simulink model "WhirlyBird_PD"  (R2016b)
settings: Solver=ode45  StartTime=0.0  StopTime=10000  RelTol=1e-3  EnableMultiTasking=on
InitFcn:
  | param
undefined symbols (not defined in the file or in its folder): drawWhirly, P, whirly_ctrl
settings Model: Creator=beard  LastModifiedBy=Jacob
settings DataIOCC: LimitDataPoints=on  SaveFormat=Array  SignalLoggingSaveFormat=ModelDataLogs
settings OptimizationCC: ExpressionDepthLimit=2147483647  InitFltsAndDblsToZero=on  LifeSpan=inf
settings DebuggingCC: UnderspecifiedInitializationDetection=Classic  MergeDetectMultiDrivingBlocksExec=none  SolverPrmCheckMsg=warning  FcnCallInpInsideContextMsg=warning  StateNameClashWarn=warning  SFUnexpectedBacktrackingDiag=warning  SFNoUnconditionalDefaultTransitionDiag=warning  SFExecutionAtInitializationDiag=none
settings HardwareCC: ProdBitPerPointer=32  ProdBitPerSizeT=32  ProdBitPerPtrDiffT=32  ProdLargestAtomicFloat=None  ProdIntDivRoundTo=Undefined  ProdEndianess=Unspecified  ProdWordSize=32  ProdHWDeviceType=32-bit Generic
settings ModelReferenceCC: PropagateSignalLabelsOutOfModel=off
settings GRTTargetCC: TargetLangStandard=C89/C90 (ANSI)  GeneratePreprocessorConditionals=Disable all  CombineOutputUpdateFcns=off  GRTInterface=on
settings ConfigComp: CovMetricSettings=dw  CovHtmlReporting=on  CovSaveCumulativeToWorkspaceVar=on  CovSaveSingleToWorkspaceVar=on  CovExternalEMLEnable=off

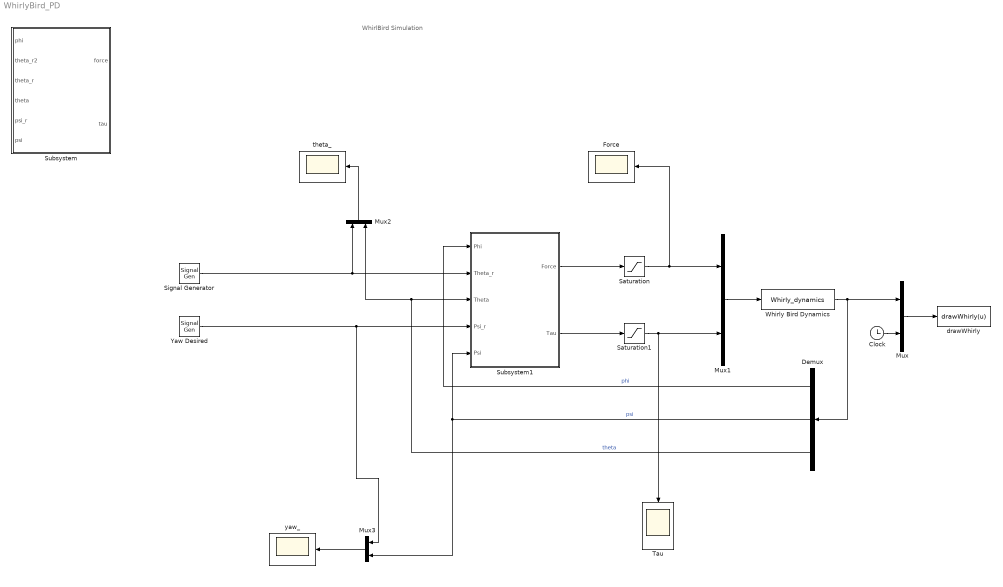
== system WhirlyBird_PD ==
  note: WhirlBird Simulation
  Clock : Clock
  Demux : Demux  Outputs=3
  Force : Scope
  Mux{,1..3} (4 alike) : Mux  Inputs=2
  Saturation : Saturate  UpperLimit=P.Fmax  LowerLimit=0
  Saturation1 : Saturate  UpperLimit=P.Taumax  LowerLimit=-P.Taumax
  Signal Generator : SignalGenerator  WaveForm=square  Amplitude=.2618*2  Frequency=.02
  Subsystem : Subsystem
  Subsystem1 : Subsystem
  Tau : Scope
  Whirly Bird Dynamics : S-Function  FunctionName=Whirly_dynamics  Parameters=P  SFunctionDeploymentMode=off  EnableBusSupport=off
  Yaw Desired : SignalGenerator  WaveForm=square  Amplitude=.2618*2  Frequency=.02
  drawWhirly : MATLABFcn  MATLABFcn=drawWhirly(u)  OutputDimensions=0  SampleTime=0.1
  theta_ : Scope
  yaw_ : Scope
  wires:
  Whirly Bird Dynamics/1 -> Mux/1, Demux/1
  Clock/1 -> Mux/2
  Mux/1 -> drawWhirly/1
  Signal Generator/1 -> Subsystem1/2(Theta_r), Mux2/1
  Mux2/1 -> theta_/1
  Mux1/1 -> Whirly Bird Dynamics/1
  Demux/3 -> Mux2/2, Subsystem1/3(Theta)  "theta"
  Saturation/1 -> Force/1, Mux1/1
  Demux/2 -> Subsystem1/5(Psi), Mux3/2  "psi"
  Yaw Desired/1 -> Mux3/1, Subsystem1/4(Psi_r)
  Mux3/1 -> yaw_/1
  Saturation1/1 -> Mux1/2, Tau/1
  Demux/1 -> Subsystem1/1(Phi)  "phi"
  Subsystem1/1(Force) -> Saturation/1
  Subsystem1/2(Tau) -> Saturation1/1

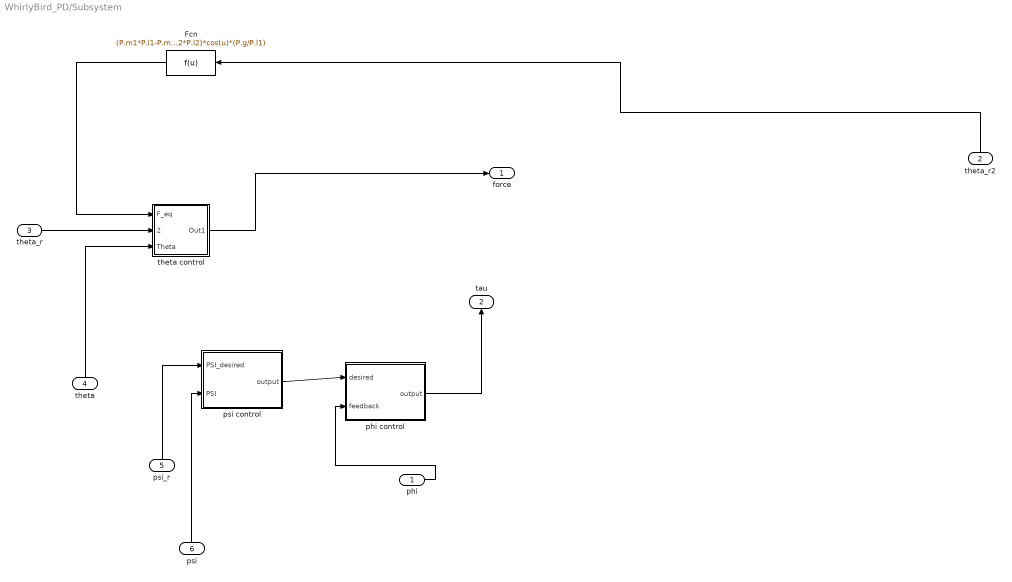
== system WhirlyBird_PD/Subsystem ==
  phi : Inport
  theta_r2 : Inport  Port=2
  theta_r : Inport  Port=3
  theta : Inport  Port=4
  psi_r : Inport  Port=5
  psi : Inport  Port=6
  Fcn : Fcn  Expr=(P.m1*P.l1-P.m2*P.l2)*cos(u)*(P.g/P.l1)
  phi control : Subsystem
  psi control : Subsystem
  theta control : Subsystem
  force : Outport
  tau : Outport  Port=2
  wires:
  theta/1 -> theta control/3(Theta)
  theta_r/1 -> theta control/2(Theta_d)
  theta_r2/1 -> Fcn/1
  psi/1 -> psi control/2(PSI)
  psi_r/1 -> psi control/1(PSI_desired)
  phi/1 -> phi control/2(feedback)
  phi control/1(output) -> tau/1
  theta control/1(Out1) -> force/1
  Fcn/1 -> theta control/1(F_eq)
  psi control/1(output) -> phi control/1(desired)

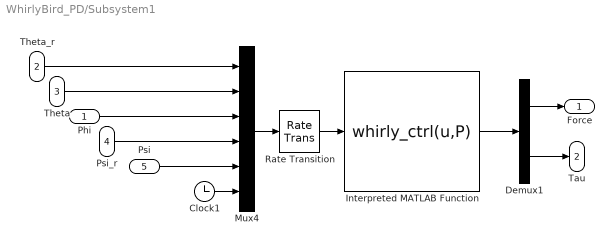
== system WhirlyBird_PD/Subsystem1 ==
  Phi : Inport
  Theta_r : Inport  Port=2
  Theta : Inport  Port=3
  Psi_r : Inport  Port=4
  Psi : Inport  Port=5
  Clock1 : Clock
  Demux1 : Demux  Outputs=2
  Interpreted MATLAB Function : MATLABFcn  MATLABFcn=whirly_ctrl(u,P)  OutputDimensions=2
  Mux4 : Mux  Inputs=6
  Rate Transition : RateTransition  OutPortSampleTime=P.Ts
  Force : Outport
  Tau : Outport  Port=2
  wires:
  Theta_r/1 -> Mux4/1
  Psi/1 -> Mux4/5
  Psi_r/1 -> Mux4/4
  Theta/1 -> Mux4/2
  Clock1/1 -> Mux4/6
  Phi/1 -> Mux4/3
  Rate Transition/1 -> Interpreted MATLAB Function/1
  Mux4/1 -> Rate Transition/1
  Interpreted MATLAB Function/1 -> Demux1/1
  Demux1/1 -> Force/1
  Demux1/2 -> Tau/1

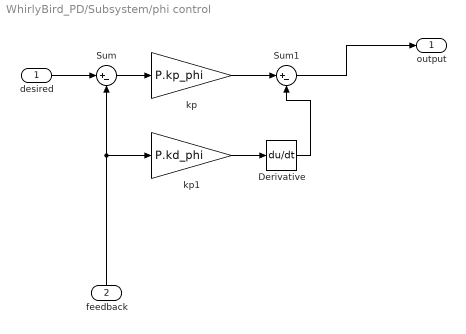
== system WhirlyBird_PD/Subsystem/phi control ==
  desired : Inport
  feedback : Inport  Port=2
  Derivative : Derivative
  Sum : Sum  Inputs=|+-
  Sum1 : Sum  Inputs=|+-
  kp : Gain  Gain=P.kp_phi
  kp1 : Gain  Gain=P.kd_phi
  output : Outport
  wires:
  desired/1 -> Sum/1
  feedback/1 -> kp1/1, Sum/2
  Sum1/1 -> output/1
  kp1/1 -> Derivative/1
  Sum/1 -> kp/1
  kp/1 -> Sum1/1
  Derivative/1 -> Sum1/2

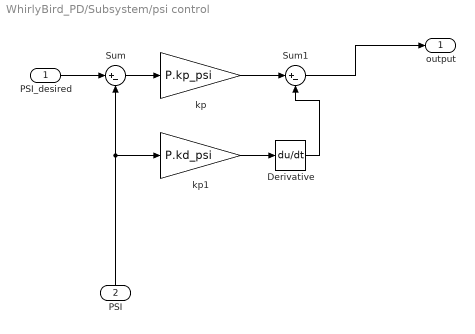
== system WhirlyBird_PD/Subsystem/psi control ==
  PSI_desired : Inport
  PSI : Inport  Port=2
  Derivative : Derivative
  Sum : Sum  Inputs=|+-
  Sum1 : Sum  Inputs=|+-
  kp : Gain  Gain=P.kp_psi
  kp1 : Gain  Gain=P.kd_psi
  output : Outport
  wires:
  PSI_desired/1 -> Sum/1
  PSI/1 -> kp1/1, Sum/2
  Sum1/1 -> output/1
  kp1/1 -> Derivative/1
  Sum/1 -> kp/1
  kp/1 -> Sum1/1
  Derivative/1 -> Sum1/2

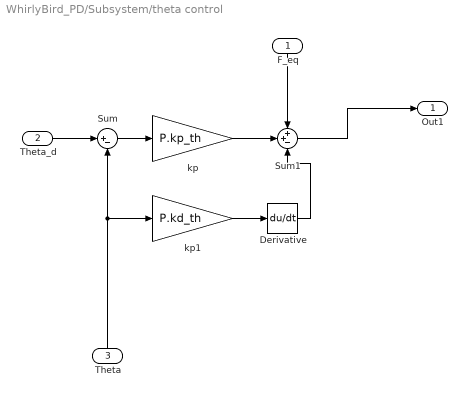
== system WhirlyBird_PD/Subsystem/theta control ==
  F_eq : Inport
  Theta_d : Inport  Port=2
  Theta : Inport  Port=3
  Derivative : Derivative
  Sum : Sum  Inputs=|+-
  Sum1 : Sum  Inputs=++-
  kp : Gain  Gain=P.kp_th
  kp1 : Gain  Gain=P.kd_th
  Out1 : Outport
  wires:
  Theta_d/1 -> Sum/1
  Theta/1 -> kp1/1, Sum/2
  kp/1 -> Sum1/2
  Sum1/1 -> Out1/1
  F_eq/1 -> Sum1/1
  Derivative/1 -> Sum1/3
  kp1/1 -> Derivative/1
  Sum/1 -> kp/1
